simulink model "ASK"  (R2021a)
settings: Solver=VariableStepAuto  StartTime=0.0  StopTime=10.0  RelTol=1e-3
libraries: commrandsrc3 x1
settings Model: Creator=Dell  LastModifiedBy=Dell

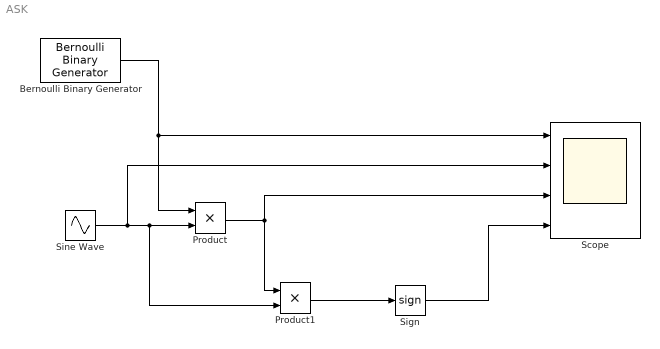
== system ASK ==
  Bernoulli Binary Generator : commrandsrc3/Bernoulli Binary Generator  ProbabilityOfZero=0.5  SeedSource=Auto  Seed=0  SampleTime=1  SamplesPerFrame=1  OutputDataType=double  SimulateUsing=Interpreted execution
  Product : Product
  Product1 : Product
  Scope : Scope  NumInputPorts=4
  Sign : Signum
  Sine Wave : Sin  Frequency=2*pi*4  SampleTime=0.01
  wires:
  Sine Wave/1 -> Scope/2, Product1/2, Product/2
  Bernoulli Binary Generator/1 -> Product/1, Scope/1
  Product/1 -> Product1/1, Scope/3
  Product1/1 -> Sign/1
  Sign/1 -> Scope/4
